simulink model "ep_10_23"  (R2023b)
settings: Solver=VariableStepAuto  StartTime=0.0  StopTime=10.0  RelTol=1e-3
libraries: cstblocks x4
settings Model: Creator=86186  LastModifiedBy=86186

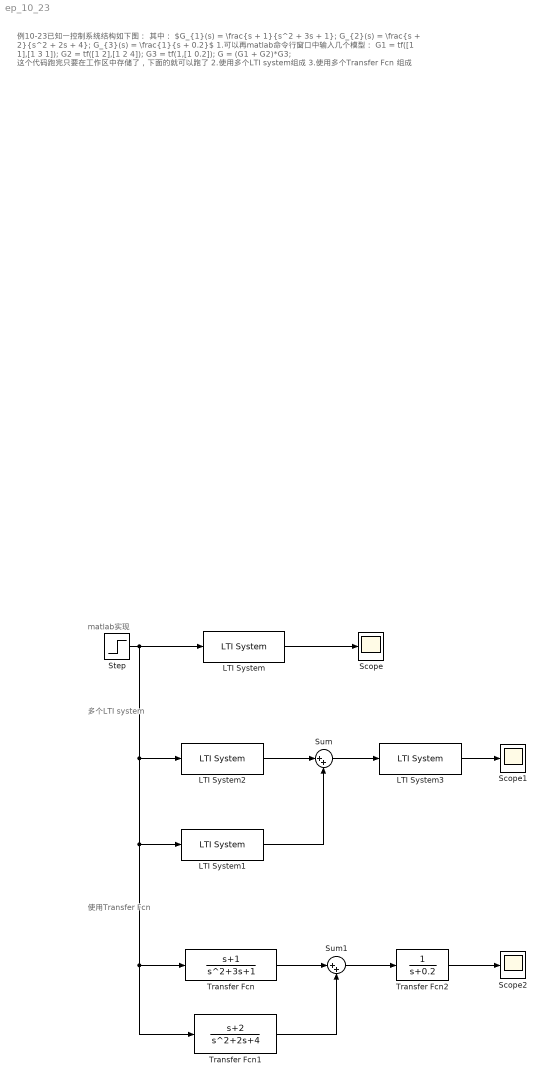
== system ep_10_23 ==
  note: 使用Transfer Fcn
  note: matlab实现
  note: 多个LTI system
  note: 例10-23已知一控制系统结构如下图：
      |
      | 其中： $G_{1}(s) = \frac{s + 1}{s^2 + 3s + 1}; G_{2}(s) = \frac{s + 2}{s^2 + 2s + 4}; G_{3}(s) = \frac{1}{s + 0.2}$
      |
      | 1.可以再matlab命令行窗口中输入几个模型：
      | G1 = tf([1 1],[1 3 1]);
      | G2 = tf([1 2],[1 2 4]);
      | G3 = tf(1,[1 0.2]);
      | G = (G1 + G2)*G3;
      | 这个代码跑完只要在工作区中存储了，下面的就可以跑了
      | 2.使用多个LTI system组成
      | 3.使用多个Transfer Fcn 组成
  LTI System : cstblocks/LTI System  sys=G  IC=[]  PadeOrder=0
  LTI System1 : cstblocks/LTI System  sys=tf([1 2],[1 2 4])  IC=[]  PadeOrder=0
  LTI System2 : cstblocks/LTI System  sys=tf([1 1],[1 3 1])  IC=[]  PadeOrder=0
  LTI System3 : cstblocks/LTI System  sys=tf(1,[1 0.2])  IC=[]  PadeOrder=0
  Scope : Scope
  Scope1 : Scope
  Scope2 : Scope
  Step : Step  SampleTime=0
  Sum : Sum  Inputs=|++
  Sum1 : Sum  Inputs=|++
  Transfer Fcn : TransferFcn  Numerator=[1 1]  Denominator=[1 3 1]
  Transfer Fcn1 : TransferFcn  Numerator=[1 2]  Denominator=[1 2 4]
  Transfer Fcn2 : TransferFcn  Denominator=[1 0.2]
  wires:
  Step/1 -> LTI System/1, LTI System2/1, Transfer Fcn1/1, Transfer Fcn/1, LTI System1/1
  LTI System/1 -> Scope/1
  LTI System2/1 -> Sum/1
  LTI System1/1 -> Sum/2
  Sum/1 -> LTI System3/1
  LTI System3/1 -> Scope1/1
  Transfer Fcn/1 -> Sum1/1
  Sum1/1 -> Transfer Fcn2/1
  Transfer Fcn1/1 -> Sum1/2
  Transfer Fcn2/1 -> Scope2/1
